simulink model "APB_Model0_v03_Test"  (R2020b)
settings: Solver=ode45  StartTime=0.0  StopTime=inf  RelTol=1e-3
undefined symbols (not defined in the file or in its folder): calb_Driver_acce, calb_Driver_bttn, calb_Driver_EmrBrk, calb_Driver_Prss, G_Fclamp, G_Kmot, G_Rmot, G_Stroke, G_SwOmega, GEN3, PbcDataStorageRequest_t
libraries: etargetslib x26, Lib_Op_Hndl x4, simulink x2, PbcOut_Checksum x2
(part 5 of 5)

== system APB_Model0_v03_Test/HstEcu/PBC/Subsystem/Subsystem4/Subsystem4 ==
  note: Invert the order of current signals. From K9 to K0
  PBCInMotorCurrentLeft_1ms : Inport
  Rate Transition : RateTransition  OutPortSampleTime=0.01
  Scope12 : Scope
  Unit Delay{18..26} (9 alike) : UnitDelay  SampleTime=0.001  HasFrameUpgradeWarning=on
  Vector Concatenate : Concatenate  NumInputs=10
  Out1 : Outport
  wires:
  Rate Transition/1 -> Out1/1
  Vector Concatenate/1 -> Rate Transition/1
  PBCInMotorCurrentLeft_1ms/1 -> Unit Delay18/1, Scope12/1, Vector Concatenate/10
  Unit Delay18/1 -> Unit Delay19/1, Vector Concatenate/9
  Unit Delay19/1 -> Unit Delay20/1, Vector Concatenate/8
  Unit Delay20/1 -> Unit Delay21/1, Vector Concatenate/7
  Unit Delay21/1 -> Unit Delay22/1, Vector Concatenate/6
  Unit Delay22/1 -> Unit Delay23/1, Vector Concatenate/5
  Unit Delay23/1 -> Unit Delay24/1, Vector Concatenate/4
  Unit Delay24/1 -> Unit Delay25/1, Vector Concatenate/3
  Unit Delay25/1 -> Unit Delay26/1, Vector Concatenate/2
  Unit Delay26/1 -> Vector Concatenate/1

== system APB_Model0_v03_Test/HstEcu/PBC/Variant Subsystem1/PFA_PBC_Gen2/Subsystem ==
  PBCInVariantItem : Inport
  Demux5 : Demux  Outputs=64
  Out1 : Outport
  wires:
  PBCInVariantItem/1 -> Demux5/1
  Demux5/1 -> Out1/1

== system APB_Model0_v03_Test/HstEcu/PBC/Variant Subsystem1/PFA_PBC_Gen3/Subsystem1 ==
  Pbc_Init : Inport  Priority=1  OutputFunctionCall=on
  Pbc_Cyclic : Inport  Priority=2  Port=2  OutputFunctionCall=on
  PbcIn : Inport  Port=3  OutDataTypeStr=Bus: PbcIn_t  BusOutputAsStruct=on
  Model : ModelReference  ModelNameDialog=SwComp_PBC  SimulationMode=Normal  ScheduleRates=on  ModelReferenceVersion=1.610
  PbcOut : Outport
  wires:
  Pbc_Init/1 -> Model/1
  PbcIn/1 -> Model/3
  Pbc_Cyclic/1 -> Model/2
  Model/1 -> PbcOut/1

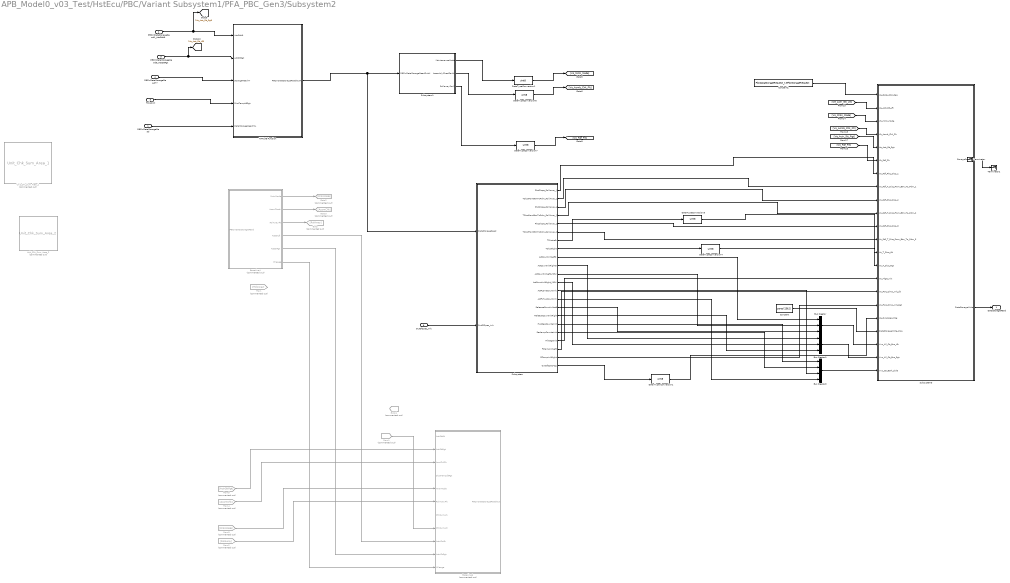
== system APB_Model0_v03_Test/HstEcu/PBC/Variant Subsystem1/PFA_PBC_Gen3/Subsystem2 ==
  PBCInDataStorageRead : Inport
      settings: AttributesFormatString=|
      | Type : %<OutDataTypeStr>
      | Unit : %<Unit>
  PBCInDataStorageRead1_ActrSttLft : Inport  Port=2
      settings: AttributesFormatString=|
      | Type : %<OutDataTypeStr>
      | Unit : %<Unit>
  PBCInDataStorageRead9_ActrSttRgt : Inport  Port=3
      settings: AttributesFormatString=|
      | Type : %<OutDataTypeStr>
      | Unit : %<Unit>
  PBCInDataStorageRead77 : Inport  Port=4
      settings: AttributesFormatString=|
      | Type : %<OutDataTypeStr>
      | Unit : %<Unit>
  TDiscInit : Inport  Port=5
      settings: AttributesFormatString=|
      | Type : %<OutDataTypeStr>
      | Unit : %<Unit>
  OutOfSpec_Init : Inport  Port=6
  BaseLine4 : MATLAB Function  Commented=on  TreatAsAtomicUnit=on
  BaseLine6 : MATLAB Function  Commented=on  TreatAsAtomicUnit=on
  Bus Creator : BusCreator  Inputs=3  OutDataTypeStr=Bus: Bus_All_Ctr  NonVirtualBus=on
      settings: InheritFromInputs=off
  Bus Creator1 : BusCreator  Inputs=3  OutDataTypeStr=Bus: Bus_All_Ctr  NonVirtualBus=on
      settings: InheritFromInputs=off
  Bus Creator2 : BusCreator  Inputs=4  OutDataTypeStr=Bus: Ctr_Both_Side  NonVirtualBus=on
      settings: InheritFromInputs=off
  Constant : Constant  Value=zeros(256,1)  OutDataTypeStr=uint8
  Constant1 : Constant  Value=PbcDataStorageRequest_t.ePbcStorageRequest  OutDataTypeStr=Enum: PbcDataStorageRequest_t
  Data Type Conversion1 : DataTypeConversion  OutDataTypeStr=uint8  SaturateOnIntegerOverflow=on  RndMeth=Zero
  DataTypeConversion{1,3..4,6..7} (5 alike) : DataTypeConversion  OutDataTypeStr=uint8  SaturateOnIntegerOverflow=on  RndMeth=Zero
  From : From  Commented=on  GotoTag=RolAway
  From1 : From  Commented=on  GotoTag=ChkAr2
  From2 : From  Commented=on  GotoTag=RolAway
  From3 : From  Commented=on  GotoTag=MntnMode
  From4 : From  Commented=on  GotoTag=AssmChk
  From5 : From  Commented=on  GotoTag=ActrSttRgt
  Goto : Goto  Commented=on  GotoTag=RolAway
  Goto1 : Goto  Commented=on  GotoTag=ChkAr2
  Goto2 : Goto  Commented=on  GotoTag=MntnMode
  Goto3 : Goto  Commented=on  GotoTag=AssmChk
  MATLAB Function : MATLAB Function  TreatAsAtomicUnit=on
  Subsystem : Subsystem
  Subsystem1 : Subsystem
  Subsystem3 : Subsystem
  Terminator : Terminator
  Terminator1 : Terminator
  Unit_Chk_Sum_Area_1 : PbcOut_Checksum/Unit_Chk_Sum_Area_1  Commented=on
      settings: SourceProductName=Hitachi SLK Library
  Unit_Chk_Sum_Area_2 : PbcOut_Checksum/Unit_Chk_Sum_Area_2  Commented=on
      settings: SourceProductName=Hitachi SLK Library
  DataStorageRead : Outport
  wires:
  BaseLine4/3(RolAwayFlt) -> Goto/1
  BaseLine4/2(AssmCheck) -> Goto3/1
  BaseLine4/1(MntnMode) -> Goto2/1
  BaseLine4/4(ActCtrLft) -> BaseLine6/9(ActnCtrLft)
  BaseLine4/5(ActCtrRgt) -> BaseLine6/10(ActnCtrRgt)
  BaseLine4/6(Mileage) -> BaseLine6/11(Mileage)
  From1/1 -> BaseLine6/8(ChkSumAr2)
  From2/1 -> BaseLine6/6(RolAwayFlt)
  From3/1 -> BaseLine6/5(MntnMode)
  From4/1 -> BaseLine6/3(AsmChkFlt)
  From5/1 -> BaseLine6/2(ActrSttRgt)
  PBCInDataStorageRead/1 -> MATLAB Function/5(DataStorageReadMIL)
  TDiscInit/1 -> MATLAB Function/4(DiscTempLftRgt)
  PBCInDataStorageRead1_ActrSttLft/1 -> MATLAB Function/1(ActrSttLft), [Ve_Actr_Stt_Rgt]
  PBCInDataStorageRead9_ActrSttRgt/1 -> [Ve_Actr_Stt_Lft], MATLAB Function/2(ActrSttRgt)
  PBCInDataStorageRead77/1 -> MATLAB Function/3(StorageRead77)
  MATLAB Function/1(PBCInDataStorageReadOutAI) -> Subsystem1/1(PBCInDataStorageReadOutAI), Subsystem/1(DataStorageRead)
  DataTypeConversion6/1 -> [Vo_Asmb_Chk_Flt]
  Subsystem/8(TDiscRight) -> DataTypeConversion4/1
  DataTypeConversion1/1 -> [Vo_Mntn_Mode]
  DataTypeConversion7/1 -> [Vo_Rdf_Flt]
  Subsystem1/3(RollawayFault) -> DataTypeConversion7/1
  Subsystem/7(TDiscLeft) -> DataTypeConversion3/1
  Subsystem1/1(MaintenanceMode) -> DataTypeConversion1/1
  Subsystem1/2(AssemblyCheckFault) -> DataTypeConversion6/1
  Subsystem/1(PbcSlope_Rollaway_1) -> Subsystem3/7(Vo_Rdf_Pbc_Slop_1)
  Subsystem/6(TDiscFromBtmToPdm_RollAway_3) -> Subsystem3/12(Vo_Rdf_T_Disc_From_Btm_To_Pdm_3)
  Subsystem/5(PbcSlope_Rollaway_3) -> Subsystem3/11(Vo_Rdf_Pbc_Slop_3)
  Subsystem/4(TDiscFromBtmToPdm_RollAway_2) -> Subsystem3/10(Vo_Rdf_T_Disc_From_Btm_To_Pdm_2)
  Subsystem/3(PbcSlope_Rollaway_2) -> Subsystem3/9(Vo_Rdf_Pbc_Slop_2)
  Subsystem/2(TDiscFromBtmToPdm_RollAway_1) -> Subsystem3/8(Vo_Rdf_T_Disc_From_Btm_To_Pdm_1)
  DataTypeConversion3/1 -> Subsystem3/13(Vo_T_Disc_Lft)
  Subsystem/22(OutOfSpecMsg) -> Data Type Conversion1/1
  OutOfSpec_Init/1 -> Subsystem/2(OutOfSpec_Init)
  [Ve_Actr_Stt_Lft] -> Subsystem3/2(Ve_Actr_Stt_Lft)
  [Vo_Rdf_Flt] -> Subsystem3/6(Vb_Rdf_Flt)
  [Ve_Actr_Stt_Rgt] -> Subsystem3/5(Ve_Actr_Stt_Rgt)
  [Vo_Asmb_Chk_Flt] -> Subsystem3/4(Vb_Asmb_Chk_Flt)
  [Vo_Mntn_Mode] -> Subsystem3/3(Vb_Mntn_Mode)
  Constant1/1 -> Subsystem3/1(Ve_Data_Stor_Req)
  DataTypeConversion4/1 -> Subsystem3/14(Vo_T_Disc_Rgt)
  Constant/1 -> Subsystem3/19(DataStorageWrite_Prev)
  Bus Creator/1 -> Subsystem3/20(Vxo_All_Ctr_Bus_Lft)
  Subsystem/9(ActCountInitLeft0) -> Bus Creator/1
  Subsystem/11(ActCountInitLeft_MGU) -> Bus Creator/2
  Subsystem/15(ReleaseCountInitLeft) -> Bus Creator/3
  Bus Creator1/1 -> Subsystem3/21(Vxo_All_Ctr_Bus_Rgt)
  Subsystem/10(ActCountInitRight0) -> Bus Creator1/1
  Subsystem/12(ActCountInitRight_MGU) -> Bus Creator1/2
  Subsystem/16(ReleaseCountInitRight) -> Bus Creator1/3
  Bus Creator2/1 -> Subsystem3/22(Vxo_Ctr_Both_Side)
  Subsystem/17(HpsReqCounterInit) -> Bus Creator2/1
  Subsystem/18(ReclampCounterInit) -> Bus Creator2/2
  Subsystem/13(ActFLOneCountInit) -> Bus Creator2/3
  Subsystem/14(ActFLTwoCountInit) -> Bus Creator2/4
  Data Type Conversion1/1 -> Subsystem3/18(Ve_Out_Spec_Msg)
  Subsystem/19(MileageInit) -> Subsystem3/15(Vo_Mlge_Init)
  Subsystem/20(FClampInitLeft) -> Subsystem3/16(Vo_Forc_Clmp_Init_Lft)
  Subsystem/21(FClampInitRight) -> Subsystem3/17(Vo_Forc_Clmp_Init_Rgt)
  Subsystem3/2("DataStorageWrite ") -> DataStorageRead/1
  Subsystem3/1(StorageRequest) -> Terminator1/1

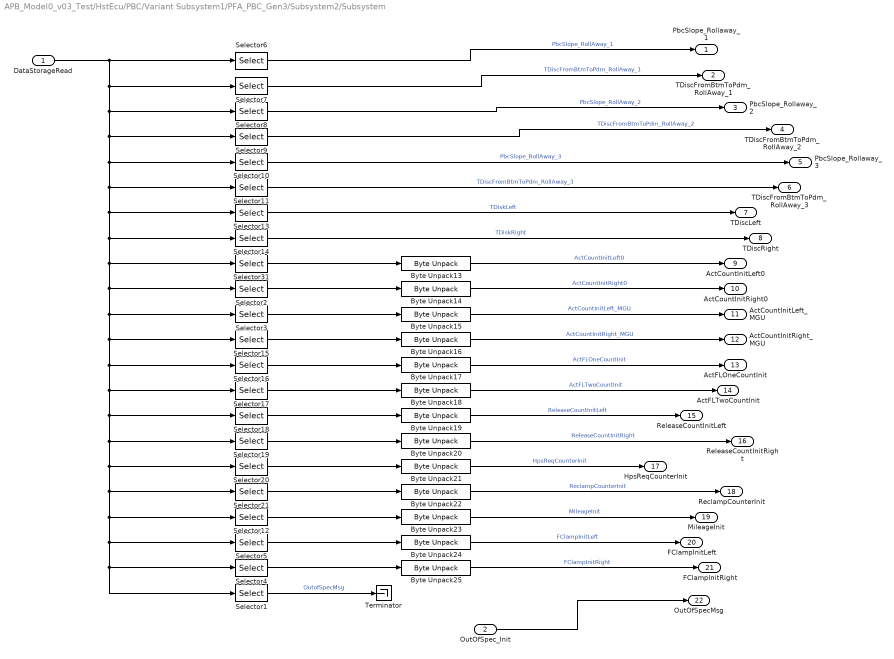
== system APB_Model0_v03_Test/HstEcu/PBC/Variant Subsystem1/PFA_PBC_Gen3/Subsystem2/Subsystem ==
  DataStorageRead : Inport
  OutOfSpec_Init : Inport  Port=2
  Byte Unpack{13..25} (13 alike) : etargetslib/Byte Unpack  dimensions={[1]}  datatypes={'uint32'}  byteAlign=1
  Selector1 : Selector  InputPortWidth=256  IndexOptions=Index vector (dialog)  Indices=[142]  OutputSizes=1
  Selector10 : Selector  InputPortWidth=256  IndexOptions=Index vector (dialog)  Indices=[65]  OutputSizes=1
  Selector11 : Selector  InputPortWidth=256  IndexOptions=Index vector (dialog)  Indices=[66]  OutputSizes=1
  Selector12 : Selector  InputPortWidth=256  IndexOptions=Index vector (dialog)  Indices=[130,131,132,133]  OutputSizes=1
  Selector13 : Selector  InputPortWidth=256  IndexOptions=Index vector (dialog)  Indices=[68]  OutputSizes=1
  Selector14 : Selector  InputPortWidth=256  IndexOptions=Index vector (dialog)  Indices=[69]  OutputSizes=1
  Selector15 : Selector  InputPortWidth=256  IndexOptions=Index vector (dialog)  Indices=[102,103,104,105]  OutputSizes=1
  Selector16 : Selector  InputPortWidth=256  IndexOptions=Index vector (dialog)  Indices=[106,107,108,109]  OutputSizes=1
  Selector17 : Selector  InputPortWidth=256  IndexOptions=Index vector (dialog)  Indices=[110,111,112,113]  OutputSizes=1
  Selector18 : Selector  InputPortWidth=256  IndexOptions=Index vector (dialog)  Indices=[114,115,116,117]  OutputSizes=1
  Selector19 : Selector  InputPortWidth=256  IndexOptions=Index vector (dialog)  Indices=[118,119,120,121]  OutputSizes=1
  Selector2 : Selector  InputPortWidth=256  IndexOptions=Index vector (dialog)  Indices=[94,95,96,97]  OutputSizes=1
  Selector20 : Selector  InputPortWidth=256  IndexOptions=Index vector (dialog)  Indices=[122,123,124,125]  OutputSizes=1
  Selector21 : Selector  InputPortWidth=256  IndexOptions=Index vector (dialog)  Indices=[126,127,128,129]  OutputSizes=1
  Selector3 : Selector  InputPortWidth=256  IndexOptions=Index vector (dialog)  Indices=[98,99,100,101]  OutputSizes=1
  Selector31 : Selector  InputPortWidth=256  IndexOptions=Index vector (dialog)  Indices=[90,91,92,93]  OutputSizes=1
  Selector4 : Selector  InputPortWidth=256  IndexOptions=Index vector (dialog)  Indices=[138,139,140,141]  OutputSizes=1
  Selector5 : Selector  InputPortWidth=256  IndexOptions=Index vector (dialog)  Indices=[134,135,136,137]  OutputSizes=1
  Selector6 : Selector  InputPortWidth=256  IndexOptions=Index vector (dialog)  Indices=[61]  OutputSizes=1
  Selector7 : Selector  InputPortWidth=256  IndexOptions=Index vector (dialog)  Indices=[62]  OutputSizes=1
  Selector8 : Selector  InputPortWidth=256  IndexOptions=Index vector (dialog)  Indices=[63]  OutputSizes=1
  Selector9 : Selector  InputPortWidth=256  IndexOptions=Index vector (dialog)  Indices=[64]  OutputSizes=1
  Terminator : Terminator
  PbcSlope_Rollaway_1 : Outport
  TDiscFromBtmToPdm_RollAway_1 : Outport  Port=2
  PbcSlope_Rollaway_2 : Outport  Port=3
  TDiscFromBtmToPdm_RollAway_2 : Outport  Port=4
  PbcSlope_Rollaway_3 : Outport  Port=5
  TDiscFromBtmToPdm_RollAway_3 : Outport  Port=6
  TDiscLeft : Outport  Port=7
  TDiscRight : Outport  Port=8
  ActCountInitLeft0 : Outport  Port=9
  ActCountInitRight0 : Outport  Port=10
  ActCountInitLeft_MGU : Outport  Port=11
  ActCountInitRight_MGU : Outport  Port=12
  ActFLOneCountInit : Outport  Port=13
  ActFLTwoCountInit : Outport  Port=14
  ReleaseCountInitLeft : Outport  Port=15
  ReleaseCountInitRight : Outport  Port=16
  HpsReqCounterInit : Outport  Port=17
  ReclampCounterInit : Outport  Port=18
  MileageInit : Outport  Port=19
  FClampInitLeft : Outport  Port=20
  FClampInitRight : Outport  Port=21
  OutOfSpecMsg : Outport  Port=22
  wires:
  Selector10/1 -> PbcSlope_Rollaway_3/1  "PbcSlope_RollAway_3"
  Byte Unpack24/1 -> FClampInitLeft/1  "FClampInitLeft"
  Byte Unpack19/1 -> ReleaseCountInitLeft/1  "ReleaseCountInitLeft"
  Byte Unpack25/1 -> FClampInitRight/1  "FClampInitRight"
  Selector13/1 -> TDiscLeft/1  "TDiskLeft"
  Selector5/1 -> Byte Unpack24/1
  Byte Unpack21/1 -> HpsReqCounterInit/1  "HpsReqCounterInit"
  Selector11/1 -> TDiscFromBtmToPdm_RollAway_3/1  "TDiscFromBtmToPdm_RollAway_3"
  Byte Unpack18/1 -> ActFLTwoCountInit/1  "ActFLTwoCountInit"
  Selector15/1 -> Byte Unpack16/1
  Selector9/1 -> TDiscFromBtmToPdm_RollAway_2/1  "TDiscFromBtmToPdm_RollAway_2"
  Selector18/1 -> Byte Unpack19/1
  Selector19/1 -> Byte Unpack20/1
  Selector3/1 -> Byte Unpack15/1
  Selector31/1 -> Byte Unpack13/1
  DataStorageRead/1 -> Selector6/1, Selector2/1, Selector3/1, Selector15/1, Selector16/1, Selector17/1, Selector18/1, Selector19/1, Selector21/1, Selector12/1, Selector5/1, Selector4/1, Selector1/1, Selector20/1, Selector31/1, Selector14/1, Selector13/1, Selector11/1, Selector10/1, Selector9/1, Selector8/1, Selector7/1
  Byte Unpack17/1 -> ActFLOneCountInit/1  "ActFLOneCountInit"
  Byte Unpack22/1 -> ReclampCounterInit/1  "ReclampCounterInit"
  Selector16/1 -> Byte Unpack17/1
  Selector7/1 -> TDiscFromBtmToPdm_RollAway_1/1  "TDiscFromBtmToPdm_RollAway_1"
  Selector12/1 -> Byte Unpack23/1
  Selector14/1 -> TDiscRight/1  "TDiskRight"
  Byte Unpack13/1 -> ActCountInitLeft0/1  "ActCountInitLeft0"
  Byte Unpack20/1 -> ReleaseCountInitRight/1  "ReleaseCountInitRight"
  Selector8/1 -> PbcSlope_Rollaway_2/1  "PbcSlope_RollAway_2"
  Byte Unpack15/1 -> ActCountInitLeft_MGU/1  "ActCountInitLeft_MGU"
  Selector20/1 -> Byte Unpack21/1
  Selector21/1 -> Byte Unpack22/1
  Byte Unpack23/1 -> MileageInit/1  "MileageInit"
  Byte Unpack14/1 -> ActCountInitRight0/1  "ActCountInitRight0"
  Selector4/1 -> Byte Unpack25/1
  Selector17/1 -> Byte Unpack18/1
  Selector6/1 -> PbcSlope_Rollaway_1/1  "PbcSlope_RollAway_1"
  Selector2/1 -> Byte Unpack14/1
  Byte Unpack16/1 -> ActCountInitRight_MGU/1  "ActCountInitRight_MGU"
  Selector1/1 -> Terminator/1  "OutofSpecMsg"
  OutOfSpec_Init/1 -> OutOfSpecMsg/1

== system APB_Model0_v03_Test/HstEcu/PBC/Variant Subsystem1/PFA_PBC_Gen3/Subsystem2/Subsystem1 ==
  PBCInDataStorageReadOutAI : Inport
  Selector1 : Selector  InputPortWidth=256  IndexOptions=Index vector (dialog)  Indices=[3]  OutputSizes=1
  Selector2 : Selector  InputPortWidth=256  IndexOptions=Index vector (dialog)  Indices=[10]  OutputSizes=1
  Selector6 : Selector  InputPortWidth=256  IndexOptions=Index vector (dialog)  Indices=[2]  OutputSizes=1
  MaintenanceMode : Outport
  AssemblyCheckFault : Outport  Port=2
  RollawayFault : Outport  Port=3
  wires:
  PBCInDataStorageReadOutAI/1 -> Selector1/1, Selector2/1, Selector6/1
  Selector6/1 -> MaintenanceMode/1
  Selector1/1 -> AssemblyCheckFault/1
  Selector2/1 -> RollawayFault/1

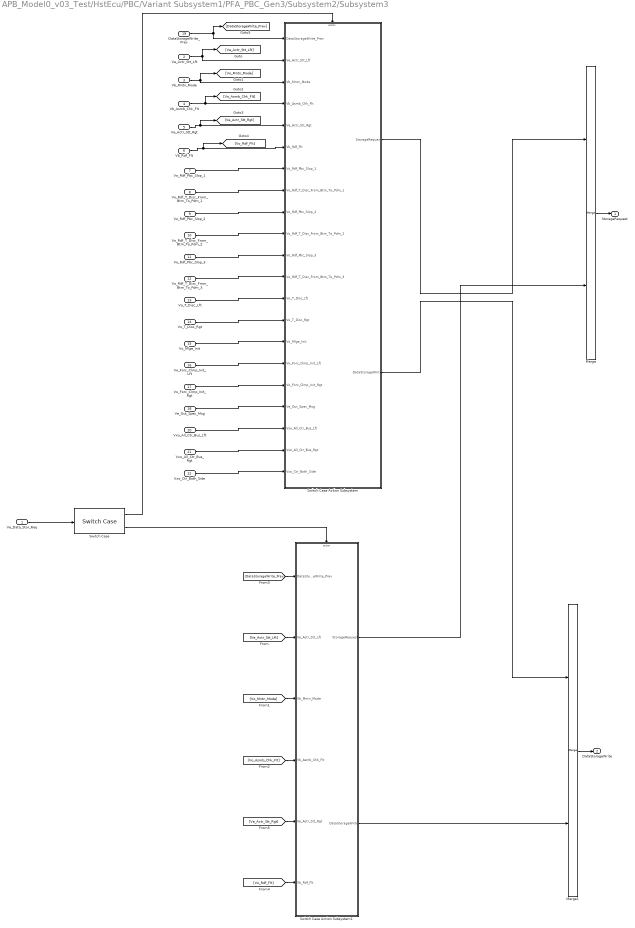
== system APB_Model0_v03_Test/HstEcu/PBC/Variant Subsystem1/PFA_PBC_Gen3/Subsystem2/Subsystem3 ==
  Ve_Data_Stor_Req : Inport
  Ve_Actr_Stt_Lft : Inport  Port=2
  Vb_Mntn_Mode : Inport  Port=3
  Vb_Asmb_Chk_Flt : Inport  Port=4
  Ve_Actr_Stt_Rgt : Inport  Port=5
  Vb_Rdf_Flt : Inport  Port=6
  Vo_Rdf_Pbc_Slop_1 : Inport  Port=7
  Vo_Rdf_T_Disc_From_Btm_To_Pdm_1 : Inport  Port=8
  Vo_Rdf_Pbc_Slop_2 : Inport  Port=9
  Vo_Rdf_T_Disc_From_Btm_To_Pdm_2 : Inport  Port=10
  Vo_Rdf_Pbc_Slop_3 : Inport  Port=11
  Vo_Rdf_T_Disc_From_Btm_To_Pdm_3 : Inport  Port=12
  Vo_T_Disc_Lft : Inport  Port=13
  Vo_T_Disc_Rgt : Inport  Port=14
  Vo_Mlge_Init : Inport  Port=15
  Vo_Forc_Clmp_Init_Lft : Inport  Port=16
  Vo_Forc_Clmp_Init_Rgt : Inport  Port=17
  Ve_Out_Spec_Msg : Inport  Port=18
  DataStorageWrite_Prev : Inport  Port=19
  Vxo_All_Ctr_Bus_Lft : Inport  Port=20
  Vxo_All_Ctr_Bus_Rgt : Inport  Port=21
  Vxo_Ctr_Both_Side : Inport  Port=22
  Merge : Merge
  Merge1 : Merge
  Switch Case : SwitchCase  CaseConditions={PbcDataStorageRequest_t.ePbcStorageRequest}
  Switch Case Action Subsystem : Subsystem  TreatAsAtomicUnit=on
  Switch Case Action Subsystem1 : Subsystem  TreatAsAtomicUnit=on
  StorageRequest : Outport
  "DataStorageWrite " : Outport  Port=2
  wires:
  Vo_Forc_Clmp_Init_Lft/1 -> Switch Case Action Subsystem/16(Vo_Forc_Clmp_Init_Lft)
  Vb_Asmb_Chk_Flt/1 -> [Vo_Asmb_Chk_Flt], Switch Case Action Subsystem/4(Vb_Asmb_Chk_Flt)
  Ve_Out_Spec_Msg/1 -> Switch Case Action Subsystem/18(Ve_Out_Spec_Msg)
  [Ve_Actr_Stt_Lft] -> Switch Case Action Subsystem1/2(Ve_Actr_Stt_Lft)
  [Vo_Rdf_Flt] -> Switch Case Action Subsystem1/6(Vb_Rdf_Flt)
  Vxo_All_Ctr_Bus_Rgt/1 -> Switch Case Action Subsystem/20(Vxo_All_Ctr_Bus_Rgt)
  Ve_Actr_Stt_Rgt/1 -> [Ve_Actr_Stt_Rgt], Switch Case Action Subsystem/5(Ve_Actr_Stt_Rgt)
  [Vo_Asmb_Chk_Flt] -> Switch Case Action Subsystem1/4(Vb_Asmb_Chk_Flt)
  DataStorageWrite_Prev/1 -> Switch Case Action Subsystem/1(DataStorageWrite_Prev), [DataStorageWrite_Prev]
  Ve_Actr_Stt_Lft/1 -> [Ve_Actr_Stt_Lft], Switch Case Action Subsystem/2(Ve_Actr_Stt_Lft)
  Vo_Rdf_T_Disc_From_Btm_To_Pdm_1/1 -> Switch Case Action Subsystem/8(Vo_Rdf_T_Disc_From_Btm_To_Pdm_1)
  Vo_Rdf_Pbc_Slop_2/1 -> Switch Case Action Subsystem/9(Vo_Rdf_Pbc_Slop_2)
  Vo_Mlge_Init/1 -> Switch Case Action Subsystem/15(Vo_Mlge_Init)
  Vo_Forc_Clmp_Init_Rgt/1 -> Switch Case Action Subsystem/17(Vo_Forc_Clmp_Init_Rgt)
  Switch Case Action Subsystem1/2("DataStorageWrite ") -> Merge1/2
  Switch Case Action Subsystem1/1(StorageRequest) -> Merge/2
  Merge/1 -> StorageRequest/1
  Switch Case/1 -> Switch Case Action Subsystem/Action
  Switch Case/2 -> Switch Case Action Subsystem1/Action
  Merge1/1 -> "DataStorageWrite "/1
  Vo_Rdf_Pbc_Slop_3/1 -> Switch Case Action Subsystem/11(Vo_Rdf_Pbc_Slop_3)
  Vb_Mntn_Mode/1 -> [Vo_Mntn_Mode], Switch Case Action Subsystem/3(Vb_Mntn_Mode)
  [DataStorageWrite_Prev] -> Switch Case Action Subsystem1/1(DataStorageWrite_Prev)
  Ve_Data_Stor_Req/1 -> Switch Case/1
  Switch Case Action Subsystem/2("DataStorageWrite ") -> Merge1/1
  Vxo_All_Ctr_Bus_Lft/1 -> Switch Case Action Subsystem/19(Vxo_All_Ctr_Bus_Lft)
  Vxo_Ctr_Both_Side/1 -> Switch Case Action Subsystem/21(Vxo_Ctr_Both_Side)
  Vo_T_Disc_Lft/1 -> Switch Case Action Subsystem/13(Vo_T_Disc_Lft)
  Vb_Rdf_Flt/1 -> [Vo_Rdf_Flt], Switch Case Action Subsystem/6(Vb_Rdf_Flt)
  Switch Case Action Subsystem/1(StorageRequest) -> Merge/1
  [Vo_Mntn_Mode] -> Switch Case Action Subsystem1/3(Vb_Mntn_Mode)
  Vo_T_Disc_Rgt/1 -> Switch Case Action Subsystem/14(Vo_T_Disc_Rgt)
  Vo_Rdf_T_Disc_From_Btm_To_Pdm_3/1 -> Switch Case Action Subsystem/12(Vo_Rdf_T_Disc_From_Btm_To_Pdm_3)
  [Ve_Actr_Stt_Rgt] -> Switch Case Action Subsystem1/5(Ve_Actr_Stt_Rgt)
  Vo_Rdf_T_Disc_From_Btm_To_Pdm_2/1 -> Switch Case Action Subsystem/10(Vo_Rdf_T_Disc_From_Btm_To_Pdm_2)
  Vo_Rdf_Pbc_Slop_1/1 -> Switch Case Action Subsystem/7(Vo_Rdf_Pbc_Slop_1)

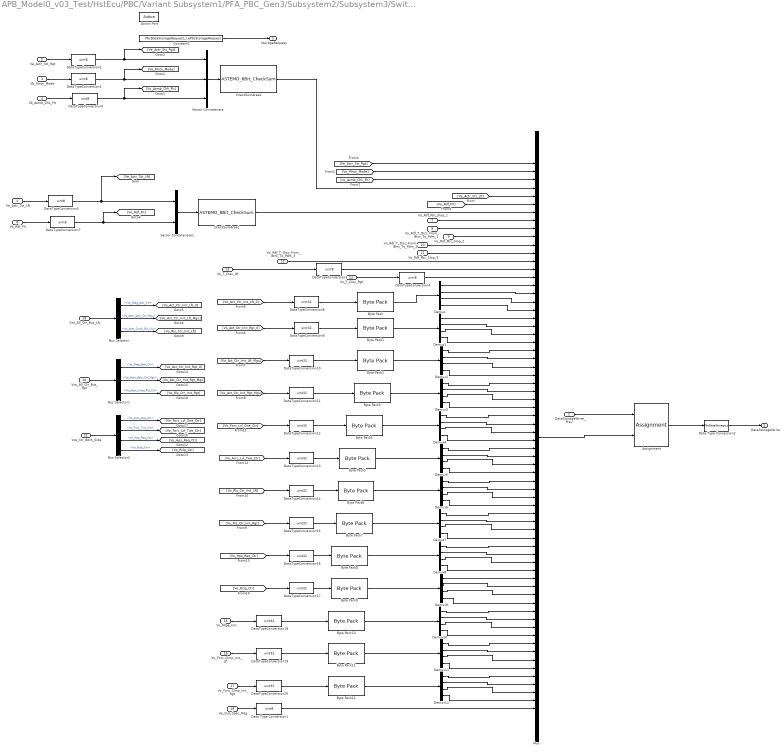
== system APB_Model0_v03_Test/HstEcu/PBC/Variant Subsystem1/PFA_PBC_Gen3/Subsystem2/Subsystem3/Switch Case Action Subsystem ==
  DataStorageWrite_Prev : Inport
  Ve_Actr_Stt_Lft : Inport  Port=2
  Vb_Mntn_Mode : Inport  Port=3
  Vb_Asmb_Chk_Flt : Inport  Port=4
  Ve_Actr_Stt_Rgt : Inport  Port=5
  Vb_Rdf_Flt : Inport  Port=6
  Vo_Rdf_Pbc_Slop_1 : Inport  Port=7
  Vo_Rdf_T_Disc_From_Btm_To_Pdm_1 : Inport  Port=8
  Vo_Rdf_Pbc_Slop_2 : Inport  Port=9
  Vo_Rdf_T_Disc_From_Btm_To_Pdm_2 : Inport  Port=10
  Vo_Rdf_Pbc_Slop_3 : Inport  Port=11
  Vo_Rdf_T_Disc_From_Btm_To_Pdm_3 : Inport  Port=12
  Vo_T_Disc_Lft : Inport  Port=13
  Vo_T_Disc_Rgt : Inport  Port=14
  Vo_Mlge_Init : Inport  Port=15
  Vo_Forc_Clmp_Init_Lft : Inport  Port=16
  Vo_Forc_Clmp_Init_Rgt : Inport  Port=17
  Ve_Out_Spec_Msg : Inport  Port=18
  Vxo_All_Ctr_Bus_Lft : Inport  Port=19
  Vxo_All_Ctr_Bus_Rgt : Inport  Port=20
  Vxo_Ctr_Both_Side : Inport  Port=21
  Action Port : ActionPort  ActionPortLabel=case [ ePbcStorageRequest ]:
  Assignment : Assignment  DiagnosticForDimensions=Warning  IndexOptions=Index vector (dialog)  Indices=[1 2 3 4 9 10 11 61 62 63 64 65 66 68 69 90 91 92 93 94 95 96 97 98 99 100 101 102 103 104 105 106 107 108 109 110 111 112 113 114 115 116 117 118 119 120 121 122 123 124 125 126 127 128 129 130 131 132 133 134 135 136 137 138 139 140 141 142]  OutputSizes=1
  Bus Selector : BusSelector  OutputSignals=Vo_Diag_Actr_Ctr,Vo_Actn_Aply_Ctr_Mgu,Vo_Actn_Cmpl_Rls_Ctr
  Bus Selector1 : BusSelector  OutputSignals=Vo_Diag_Actr_Ctr,Vo_Actn_Aply_Ctr_Mgu,Vo_Actn_Cmpl_Rls_Ctr
  Bus Selector2 : BusSelector  OutputSignals=Vo_Forc_One_Ctr,Vo_Forc_Two_Ctr,Vo_Hps_Req_Ctr,Vo_Rclp_Ctr
  Byte Pack{,1..12} (13 alike) : etargetslib/Byte Pack  datatypes={'uint32'}  byteAlign=1
  CheckSumArea1 : Lib_Op_Hndl/ASTEMO_8Bit_CheckSum
  CheckSumArea2 : Lib_Op_Hndl/ASTEMO_8Bit_CheckSum
  Constant1 : Constant  Value=PbcDataStorageRequest_t.ePbcStorageRequest  OutDataTypeStr=Enum: PbcDataStorageRequest_t
  Data Type Conversion1 : DataTypeConversion  OutDataTypeStr=uint8  SaturateOnIntegerOverflow=on  RndMeth=Zero
  Data Type Conversion2 : DataTypeConversion  OutDataTypeStr=PbcDataStorage_t
  DataTypeConversion{1..7} (7 alike) : DataTypeConversion  OutDataTypeStr=uint8  SaturateOnIntegerOverflow=on  RndMeth=Zero
  DataTypeConversion{8..20} (13 alike) : DataTypeConversion  OutDataTypeStr=uint32  SaturateOnIntegerOverflow=on  RndMeth=Zero
  Demux{,1..12} (13 alike) : Demux
  Mux : Mux  Inputs=68
  Vector Concatenate : Concatenate  NumInputs=3
  Vector Concatenate1 : Concatenate
  StorageRequest : Outport
  "DataStorageWrite " : Outport  Port=2
  wires:
  Constant1/1 -> StorageRequest/1
  [Vo_Rls_Ctr_Init_Lft] -> DataTypeConversion14/1
  Vo_Mlge_Init/1 -> DataTypeConversion18/1
  Vo_Forc_Clmp_Init_Rgt/1 -> DataTypeConversion20/1
  Vo_Forc_Clmp_Init_Lft/1 -> DataTypeConversion19/1
  [Vo_Act_Ctr_Init_Lft_Mgu] -> DataTypeConversion10/1
  CheckSumArea2/1 -> Mux/4
  [Vo_Asmb_Chk_Flt] -> Mux/3
  Data Type Conversion2/1 -> "DataStorageWrite "/1
  DataStorageWrite_Prev/1 -> Assignment/1
  [Ve_Actr_Stt_Rgt] -> Mux/1
  Assignment/1 -> Data Type Conversion2/1
  [Vo_Mntn_Mode] -> Mux/2
  CheckSumArea1/1 -> Mux/7
  Vb_Asmb_Chk_Flt/1 -> DataTypeConversion6/1
  Ve_Out_Spec_Msg/1 -> Data Type Conversion1/1
  DataTypeConversion7/1 -> Vector Concatenate1/2, [Vo_Rdf_Flt]
  Vo_Rdf_T_Disc_From_Btm_To_Pdm_1/1 -> Mux/9
  DataTypeConversion3/1 -> Mux/14
  Vo_T_Disc_Rgt/1 -> DataTypeConversion4/1
  Vector Concatenate/1 -> CheckSumArea2/1
  Ve_Actr_Stt_Lft/1 -> DataTypeConversion5/1
  Vo_Rdf_T_Disc_From_Btm_To_Pdm_3/1 -> Mux/13
  Vo_Rdf_Pbc_Slop_3/1 -> Mux/12
  Vo_Rdf_T_Disc_From_Btm_To_Pdm_2/1 -> Mux/11
  Vb_Rdf_Flt/1 -> DataTypeConversion7/1
  Vo_T_Disc_Lft/1 -> DataTypeConversion3/1
  DataTypeConversion1/1 -> Vector Concatenate/2, [Vo_Mntn_Mode]
  DataTypeConversion2/1 -> Vector Concatenate/1, [Ve_Actr_Stt_Rgt]
  Demux2/2 -> Mux/25
  Demux1/1 -> Mux/20
  Demux1/4 -> Mux/23
  Data Type Conversion1/1 -> Mux/68
  Demux2/1 -> Mux/24
  DataTypeConversion4/1 -> Mux/15
  [Ve_Actr_Stt_Lft] -> Mux/5
  Vo_Rdf_Pbc_Slop_1/1 -> Mux/8
  Vb_Mntn_Mode/1 -> DataTypeConversion1/1
  DataTypeConversion6/1 -> Vector Concatenate/3, [Vo_Asmb_Chk_Flt]
  Vo_Rdf_Pbc_Slop_2/1 -> Mux/10
  DataTypeConversion5/1 -> Vector Concatenate1/1, [Ve_Actr_Stt_Lft]
  [Vo_Rdf_Flt] -> Mux/6
  Vector Concatenate1/1 -> CheckSumArea1/1
  Ve_Actr_Stt_Rgt/1 -> DataTypeConversion2/1
  Demux2/3 -> Mux/26
  Byte Pack4/1 -> Demux4/1
  Byte Pack3/1 -> Demux3/1
  Byte Pack5/1 -> Demux5/1
  Mux/1 -> Assignment/2
  Byte Pack2/1 -> Demux2/1
  Byte Pack11/1 -> Demux11/1
  Byte Pack12/1 -> Demux12/1
  DataTypeConversion15/1 -> Byte Pack7/1
  Demux1/3 -> Mux/22
  DataTypeConversion13/1 -> Byte Pack5/1
  DataTypeConversion12/1 -> Byte Pack4/1
  DataTypeConversion10/1 -> Byte Pack2/1
  Demux/4 -> Mux/19
  Byte Pack/1 -> Demux/1
  Demux/3 -> Mux/18
  Demux/2 -> Mux/17
  Demux12/1 -> Mux/64
  Demux10/2 -> Mux/57
  Demux/1 -> Mux/16
  Demux11/3 -> Mux/62
  Demux12/4 -> Mux/67
  Demux12/3 -> Mux/66
  DataTypeConversion20/1 -> Byte Pack12/1
  Demux11/4 -> Mux/63
  Byte Pack1/1 -> Demux1/1
  DataTypeConversion19/1 -> Byte Pack11/1
  Demux11/1 -> Mux/60
  DataTypeConversion17/1 -> Byte Pack9/1
  Demux8/2 -> Mux/49
  Demux9/3 -> Mux/54
  Demux7/2 -> Mux/45
  Demux7/3 -> Mux/46
  Demux12/2 -> Mux/65
  Demux8/4 -> Mux/51
  Demux8/3 -> Mux/50
  Demux9/4 -> Mux/55
  Demux8/1 -> Mux/48
  Demux7/1 -> Mux/44
  Demux10/1 -> Mux/56
  Demux7/4 -> Mux/47
  Byte Pack6/1 -> Demux6/1
  Byte Pack10/1 -> Demux10/1
  DataTypeConversion16/1 -> Byte Pack8/1
  Demux5/1 -> Mux/36
  Demux5/2 -> Mux/37
  Byte Pack7/1 -> Demux7/1
  Demux5/4 -> Mux/39
  Demux4/3 -> Mux/34
  Demux4/4 -> Mux/35
  Byte Pack8/1 -> Demux8/1
  Demux4/2 -> Mux/33
  DataTypeConversion18/1 -> Byte Pack10/1
  Demux4/1 -> Mux/32
  Demux10/3 -> Mux/58
  Demux3/1 -> Mux/28
  DataTypeConversion11/1 -> Byte Pack3/1
  [Vo_Forc_Lvl_One_Ctr] -> DataTypeConversion12/1
  Demux6/1 -> Mux/40
  Demux6/3 -> Mux/42
  Demux3/3 -> Mux/30
  Demux9/1 -> Mux/52
  DataTypeConversion14/1 -> Byte Pack6/1
  Demux6/4 -> Mux/43
  Demux10/4 -> Mux/59
  Demux3/2 -> Mux/29
  Demux2/4 -> Mux/27
  DataTypeConversion9/1 -> Byte Pack1/1
  Demux6/2 -> Mux/41
  Byte Pack9/1 -> Demux9/1
  Demux5/3 -> Mux/38
  Demux11/2 -> Mux/61
  Demux9/2 -> Mux/53
  Demux3/4 -> Mux/31
  DataTypeConversion8/1 -> Byte Pack/1
  Demux1/2 -> Mux/21
  Vxo_All_Ctr_Bus_Lft/1 -> Bus Selector/1
  Vxo_All_Ctr_Bus_Rgt/1 -> Bus Selector1/1
  [Vo_Act_Ctr_Init_Lft_0] -> DataTypeConversion8/1
  [Vo_Act_Ctr_Init_Rgt_0] -> DataTypeConversion9/1
  [Vo_Act_Ctr_Init_Rgt_Mgu] -> DataTypeConversion11/1
  [Vo_Rls_Ctr_Init_Rgt] -> DataTypeConversion15/1
  [Vo_Forc_Lvl_Two_Ctr] -> DataTypeConversion13/1
  [Vo_Hps_Req_Ctr] -> DataTypeConversion16/1
  [Vo_Rclp_Ctr] -> DataTypeConversion17/1
  Bus Selector/3 -> [Vo_Rls_Ctr_Init_Lft]  "<Vo_Actn_Cmpl_Rls_Ctr>"
  Bus Selector/2 -> [Vo_Act_Ctr_Init_Lft_Mgu]  "<Vo_Actn_Aply_Ctr_Mgu>"
  Bus Selector/1 -> [Vo_Act_Ctr_Init_Lft_0]  "<Vo_Diag_Actr_Ctr>"
  Bus Selector1/2 -> [Vo_Act_Ctr_Init_Rgt_Mgu]  "<Vo_Actn_Aply_Ctr_Mgu>"
  Bus Selector1/3 -> [Vo_Rls_Ctr_Init_Rgt]  "<Vo_Actn_Cmpl_Rls_Ctr>"
  Bus Selector1/1 -> [Vo_Act_Ctr_Init_Rgt_0]  "<Vo_Diag_Actr_Ctr>"
  Vxo_Ctr_Both_Side/1 -> Bus Selector2/1
  Bus Selector2/1 -> [Vo_Forc_Lvl_One_Ctr]  "<Vo_Forc_One_Ctr>"
  Bus Selector2/2 -> [Vo_Forc_Lvl_Two_Ctr]  "<Vo_Forc_Two_Ctr>"
  Bus Selector2/3 -> [Vo_Hps_Req_Ctr]  "<Vo_Hps_Req_Ctr>"
  Bus Selector2/4 -> [Vo_Rclp_Ctr]  "<Vo_Rclp_Ctr>"

== system APB_Model0_v03_Test/HstEcu/PBC/Variant Subsystem1/PFA_PBC_Gen3/Subsystem2/Subsystem3/Switch Case Action Subsystem1 ==
  DataStorageWrite_Prev : Inport
  Ve_Actr_Stt_Lft : Inport  Port=2
  Vb_Mntn_Mode : Inport  Port=3
  Vb_Asmb_Chk_Flt : Inport  Port=4
  Ve_Actr_Stt_Rgt : Inport  Port=5
  Vb_Rdf_Flt : Inport  Port=6
  Action Port : ActionPort  ActionPortLabel=default:
  Assignment : Assignment  DiagnosticForDimensions=Warning  IndexOptions=Index vector (dialog)  Indices=[1 2 3 4 9 10 11]  OutputSizes=1
  CheckSumArea1 : Lib_Op_Hndl/ASTEMO_8Bit_CheckSum
  CheckSumArea2 : Lib_Op_Hndl/ASTEMO_8Bit_CheckSum
  Constant2 : Constant  Value=PbcDataStorageRequest_t.ePbcNoStorageRequest  OutDataTypeStr=Enum: PbcDataStorageRequest_t
  Data Type Conversion2 : DataTypeConversion  OutDataTypeStr=PbcDataStorage_t
  DataTypeConversion{1..2,5..7} (5 alike) : DataTypeConversion  OutDataTypeStr=uint8  SaturateOnIntegerOverflow=on  RndMeth=Zero
  Mux : Mux  Inputs=7
  Vector Concatenate : Concatenate  NumInputs=3
  Vector Concatenate1 : Concatenate
  StorageRequest : Outport
  "DataStorageWrite " : Outport  Port=2
  wires:
  Constant2/1 -> StorageRequest/1
  CheckSumArea2/1 -> Mux/4
  [Vo_Asmb_Chk_Flt] -> Mux/3
  Data Type Conversion2/1 -> "DataStorageWrite "/1
  DataStorageWrite_Prev/1 -> Assignment/1
  [Ve_Actr_Stt_Rgt] -> Mux/1
  Assignment/1 -> Data Type Conversion2/1
  [Vo_Mntn_Mode] -> Mux/2
  CheckSumArea1/1 -> Mux/7
  Vb_Asmb_Chk_Flt/1 -> DataTypeConversion6/1
  DataTypeConversion7/1 -> Vector Concatenate1/2, [Vo_Rdf_Flt]
  Vector Concatenate/1 -> CheckSumArea2/1
  Ve_Actr_Stt_Lft/1 -> DataTypeConversion5/1
  Vb_Rdf_Flt/1 -> DataTypeConversion7/1
  DataTypeConversion1/1 -> Vector Concatenate/2, [Vo_Mntn_Mode]
  DataTypeConversion2/1 -> Vector Concatenate/1, [Ve_Actr_Stt_Rgt]
  [Ve_Actr_Stt_Lft] -> Mux/5
  Vb_Mntn_Mode/1 -> DataTypeConversion1/1
  DataTypeConversion6/1 -> Vector Concatenate/3, [Vo_Asmb_Chk_Flt]
  DataTypeConversion5/1 -> Vector Concatenate1/1, [Ve_Actr_Stt_Lft]
  [Vo_Rdf_Flt] -> Mux/6
  Vector Concatenate1/1 -> CheckSumArea1/1
  Ve_Actr_Stt_Rgt/1 -> DataTypeConversion2/1
  Mux/1 -> Assignment/2

== matlab function APB_Model0_v03_Test/HstEcu/PBC/Variant Subsystem1/PFA_PBC_Gen3/MATLAB Function2 ==
  data: PBCOutDataStorageWrite input; PBCOutDataStorageWrite_MIL output
function PBCOutDataStorageWrite_MIL  = fcn_2(PBCOutDataStorageWrite)
PBCOutDataStorageWrite_MIL =linspace(0,0,251) ;

for i=2:8
    PBCOutDataStorageWrite_MIL(i-1) = PBCOutDataStorageWrite(i) ;
end
for i=10:76
    PBCOutDataStorageWrite_MIL(i-2) = PBCOutDataStorageWrite(i) ;
end
PBCOutDataStorageWrite_MIL(75) = PBCOutDataStorageWrite(78) ;
PBCOutDataStorageWrite_MIL(76) = PBCOutDataStorageWrite(79) ;

for i=82:256
    PBCOutDataStorageWrite_MIL(i-5) = PBCOutDataStorageWrite(i) ;
end
end

== matlab function APB_Model0_v03_Test/HstEcu/PBC/Variant Subsystem1/PFA_PBC_Gen3/MATLAB Function3 ==
  data: u input; y output
function y = mapping(u)

if u==1
y = uint8(27);
else if u==2
        y=uint8(40) ;
    else if u==3
        y=uint8(54) ;
        else if u==4
        y=uint8(113) ;
        else if u==5
        y=uint8(142) ;
        else if u==6
        y=uint8(144) ;
        else if u==7
        y=uint8(163) ;
        else if u==8
        y=uint8(189) ;
            
            else y = (u) ;
            end
            end
            end
            end
            end
            end
            end
        end
    end

== stateflow chart APB_Model0_v03_Test/HstEcu/Chart1 ==
  settings: sampleTime=0.001
  state PBCInitialize
    en:
    sc=0;
    HostCall, Init;
    du:
    sc=0;
    HostCall, Init;
    In=0;
  state Host1
    en:
    if (sc~=-1)
    HostCall
    end
    sc=sc+1;
    In=In+1;
    du:
    HostCall;
    sc=sc+1;
    In=In+1;
    end
  state PBC1
    en:
    In=0;
    HostCall, Step;
    sc=0;
    du:
    HostCall, Step ;
    sc=0;
  Host1 -> PBCInitialize [order 2] : [sc==9 && In==11]
  PBCInitialize -> Host1 : [sc==0]
  (default) -> Host1 : {sc= -1, In= 1; HostCall;}
  PBC1 -> Host1 : [sc==0 ]
  Host1 -> PBC1 [order 1] : [sc==9 && In~=11]
  data: sc local =0; In local
  events: HostCall output FUNCTION_CALL_EVENT; Init output FUNCTION_CALL_EVENT; Step output FUNCTION_CALL_EVENT; Samp input FUNCTION_CALL_EVENT

== matlab function APB_Model0_v03_Test/HstEcu/PBC/Variant Subsystem1/PFA_PBC_Gen3/Subsystem2/BaseLine4 ==
  data: PBCInDataStorageRead input; MntnMode output; AssmCheck output; RolAwayFlt output; ActCtrLft output; ActCtrRgt output; Mileage output
function [MntnMode, AssmCheck, RolAwayFlt, ActCtrLft, ActCtrRgt, Mileage ] = fcn(PBCInDataStorageRead)
MntnMode = PBCInDataStorageRead(2); % 2 in data 
AssmCheck =  PBCInDataStorageRead(3); % 3 in data
RolAwayFlt = PBCInDataStorageRead(10); % 10 in data
ActCtrLft = PBCInDataStorageRead(90:93); % 90 : 93 in data -> 1, 9 , 77 to be removed 
ActCtrRgt = PBCInDataStorageRead(94:97); % 94 : 97
Mileage = PBCInDataStorageRead(130:133); % 130 : 133
end

== matlab function APB_Model0_v03_Test/HstEcu/PBC/Variant Subsystem1/PFA_PBC_Gen3/Subsystem2/BaseLine6 ==
  data: PBCInDataStorageReadOut output; ActrSttLft input; ActrSttRgt input; AsmChkFlt input; DiscTempLftRgt input; MntnMode input; RolAwayFlt input; ChkSumAr1 input; ChkSumAr2 input; ActnCtrLft input; ActnCtrRgt input; Mileage input
function PBCInDataStorageReadOut = fcn(ActrSttLft, ActrSttRgt, AsmChkFlt, DiscTempLftRgt,MntnMode,RolAwayFlt, ChkSumAr1, ChkSumAr2, ActnCtrLft, ActnCtrRgt, Mileage)

% Initialise PBCInDataStorageReadOut
PBCInDataStorageReadOut = uint8(zeros(256, 1));


% Assign Bytes
% Area 1
PBCInDataStorageReadOut(1) = ActrSttLft;
PBCInDataStorageReadOut(2) = MntnMode;
PBCInDataStorageReadOut(3) = AsmChkFlt;
PBCInDataStorageReadOut(4) = ChkSumAr2;

% Area 2
PBCInDataStorageReadOut(9) = ActrSttRgt;
PBCInDataStorageReadOut(10) = RolAwayFlt;
PBCInDataStorageReadOut(11) = ChkSumAr1;

% Area 3
PBCInDataStorageReadOut(68) = DiscTempLftRgt;
PBCInDataStorageReadOut(69) = DiscTempLftRgt;
PBCInDataStorageReadOut(90:93) = ActnCtrLft;
PBCInDataStorageReadOut(94:97) = ActnCtrRgt;
PBCInDataStorageReadOut(130:133) = Mileage;
end

== matlab function APB_Model0_v03_Test/HstEcu/PBC/Variant Subsystem1/PFA_PBC_Gen3/Subsystem2/MATLAB Function ==
  data: ActrSttLft input; PBCInDataStorageReadOutAI output; ActrSttRgt input; StorageRead77 input; DiscTempLftRgt input; DataStorageReadMIL input
function PBCInDataStorageReadOutAI = fcn(ActrSttLft, ActrSttRgt, StorageRead77, DiscTempLftRgt,DataStorageReadMIL)

% Initialise PBCInDataStorageReadOut
PBCInDataStorageReadOutAI = uint8(zeros(256, 1));


% Assign Bytes
% Area 1
PBCInDataStorageReadOutAI(1) = ActrSttLft;
PBCInDataStorageReadOutAI(2:8) = DataStorageReadMIL(1:7);

% Area 2
PBCInDataStorageReadOutAI(9) = ActrSttRgt;
PBCInDataStorageReadOutAI(10:67) = DataStorageReadMIL(8:65);

% Area 3
PBCInDataStorageReadOutAI(68) = DiscTempLftRgt;
PBCInDataStorageReadOutAI(69) = DiscTempLftRgt;
PBCInDataStorageReadOutAI(70:76) = DataStorageReadMIL(66:72);
PBCInDataStorageReadOutAI(77) = StorageRead77 ;
PBCInDataStorageReadOutAI(78:256) = DataStorageReadMIL(73:251);

end

== matlab function APB_Model0_v03_Test/HstEcu/PBC/Variant Subsystem1/PFA_PBC_Gen3/MATLAB Function ==
  data: u input; y output
function y = mapping(u)

if u==1
y = uint8(27);
else if u==2
        y=uint8(40) ;
    else if u==3
        y=uint8(54) ;
        else if u==4
        y=uint8(113) ;
        else if u==5
        y=uint8(142) ;
        else if u==6
        y=uint8(144) ;
        else if u==7
        y=uint8(163) ;
        else if u==8
        y=uint8(189) ;
            
            else y = (u) ;
            end
            end
            end
            end
            end
            end
            end
        end
    end

== matlab function APB_Model0_v03_Test/HstEcu/PBC/Variant Subsystem1/PFA_PBC_Gen3/MATLAB Function1 ==
  data: PBCOutDataStorageWrite input; PBCOutDataStorageWrite1 output; PBCOutDataStorageWrite9 output; PBCOutDataStorageWrite77 output; PBCOutDataStorageWrite80 output; PBCOutDataStorageWrite81 output
function [PBCOutDataStorageWrite1, PBCOutDataStorageWrite9, PBCOutDataStorageWrite77, PBCOutDataStorageWrite80, PBCOutDataStorageWrite81] = fcn(PBCOutDataStorageWrite)

PBCOutDataStorageWrite1 = double(PBCOutDataStorageWrite(1));
PBCOutDataStorageWrite9 = double(PBCOutDataStorageWrite(9));
PBCOutDataStorageWrite77 = double(PBCOutDataStorageWrite(77));
PBCOutDataStorageWrite80 = double(PBCOutDataStorageWrite(80));
PBCOutDataStorageWrite81 = double(PBCOutDataStorageWrite(81));
end
